simulink model "BLAC_MotorCtrl_Math"  (R2025b)
settings: Solver=FixedStepDiscrete  StartTime=0.0  StopTime=5  FixedStep=MC_Sim_BaseStep  RelTol=1e-3  EnableMultiTasking=on
values from neighbouring files (symbols this model uses):
  MC_Hardware_Chip_ADCResultBit = 0.0    [MotorControlDataDictionary_Math.sldd]
  MC_Hardware_Chip_ADCVoltageMax = 1.0    [MotorControlDataDictionary_Math.sldd]
  MC_Hardware_Chip_ADCVoltageRefence = 0.0    [MotorControlDataDictionary_Math.sldd]
  MC_Hardware_Chip_CSAGain = 1.0    [MotorControlDataDictionary_Math.sldd]
  MC_Sim_BaseStep = 2.5E-8    [MotorControlDataDictionary_Math.sldd]
  MC_Sim_HFTStep = 6.6675E-5    [MotorControlDataDictionary_Math.sldd]
undefined symbols (not defined in the file or in its folder): MC_MOS_DeadTime, MC_Motor_Phi, MC_Motor_Rotor_Pn, MC_Motor_Stator_Ld, MC_Motor_Stator_Lq, MC_Motor_Stator_Rs, MC_Param_CurrentPI_Ki, MC_Param_CurrentPI_Kp, MC_Param_CurrentPI_UdInteMax, MC_Param_CurrentPI_UdInteMin, MC_Param_CurrentPI_UdMax, MC_Param_CurrentPI_UdMin, MC_Param_CurrentPI_UqInteMax, MC_Param_CurrentPI_UqInteMin, MC_Param_CurrentPI_UqMax, MC_Param_CurrentPI_UqMin, MC_Param_Flux_Gamma, MC_Param_Flux_Lalpha, MC_Param_Flux_Lbeta, MC_Param_Flux_Ralpha, MC_Param_Flux_Rbeta, MC_Param_Luen_BEMFalpha, MC_Param_Luen_BEMFbeta, MC_Param_Luen_BEMFErr, MC_Param_Luen_Currentalpha, MC_Param_Luen_Currentbeta, MC_Param_Luen_CurrentErr, MC_Param_Luen_PLL_Ki, MC_Param_Luen_PLL_Kp, MC_Param_Luen_Voltagealpha, MC_Param_Luen_Voltagebeta, MC_Param_PhasetoReal, MC_Param_SMO_CoffA, MC_Param_SMO_CoffB, MC_Param_SpeedtoTheta, MC_Param_SVPWM_DutyMax, MC_Param_SVPWM_DutyMin, MC_Param_SVPWM_SampleOffset1, MC_Param_SVPWM_SampleOffset2, MC_Param_SVPWM_SampleValid
libraries: simulink x31, nesl_utility x22, ee_lib x21, fl_lib x16, spsSeriesRLCBranchLib x2, spsVoltageMeasurementLib x2
(part 3 of 5)

== system BLAC_MotorCtrl_Math/Hardware_Sim/IGBT_Inverter_Sim ==
  DriveA : Inport
  DriveB : Inport  Port=2
  DriveC : Inport  Port=3
  Demux : Demux  Outputs=2
  Demux1 : Demux  Outputs=2
  Demux2 : Demux  Outputs=2
  IGBT_AH : ee_lib/Semiconductors & Converters/IGBT (Ideal, Switching)  port_option=ee.enum.controlport.ps  Vf=0.8 V  Ron=0.001 Ohm  Goff=1e-5 1/Ohm  Vth=6 V  diode_param=ee.enum.semiconductors.protectionDiode.external  diode_Vf=0.8 V  diode_Ron=0.001 Ohm  diode_Goff=1e-5 1/Ohm  diode_C=50e-9 F  diode_iRM=-235 A  diode_iF=300 A  diode_idot=-50 A/us  diode_trr_param=ee.enum.converters.diodeReverseParam.trr_factor  diode_trr_factor=3  diode_trr=15 us  diode_Qrr=1500 s*uA  ice_specify=off  ice_priority=None  ice=0 A  ice_nominal_specify=off  ice_nominal_value=1  ice_nominal_unit=A  vce_specify=off  vce_priority=None  vce=0 V  vce_nominal_specify=off  vce_nominal_value=1  vce_nominal_unit=V  vge_specify=off  vge_priority=None  vge=0 V  vge_nominal_specify=off  vge_nominal_value=1  vge_nominal_unit=V  thermal_loss_option=ee.enum.converters.thermalLossOption.constantvalues  Von_data=[0, .1, .6, .8, 1, 1.3, 1.6, 2, 2.4; 0, .1, .7, 1, 1.2, 1.5, 1.9, 2.4, 2.8] V  Tj=[298.15, 398.15] K  Iout_data=[0, .1, 1, 5, 10, 20, 40, 70, 100] A  Eon_data=[0, .0024, .024, .12, .2, .48, 1.04, 2.16, 3.24; 0, .003, .03, .15, .25, .6, 1.3, 2.7, 4.05] * 1e-3 J  Eoff_data=[0, .0007, .0066, .033, .066, .17, .33, .83, 1.5; 0, .001, .01, .05, .1, .25, .5, 1.2, 2.2] * 1e-3 J  Eon_data_3D=[zeros(2, 9, 3)] J  Eoff_data_3D=[zeros(2, 9, 3)] J  Tj_loss=[298.15, 398.15] K  Iout_data_loss=[0, .1, 1, 5, 10, 20, 40, 70, 100] A  tabulateWithVce=false  Vce_loss=[0, 150, 300] V  Eon_scalar=22.86e-3 J  Eoff_scalar=17.14e-3 J  Voff=300 V  Iout_scalar=600 A  useCurrentFromPreviousCycle=false  useVoltageFromPreviousCycle=false  diodeModelType=ee.enum.converters.diodeModelType.pwl  diodeTableType=ee.enum.diode.tableType.IfMat  diode_ReverseIVType=ee.enum.diode.diodeReverseIV.constant  diode_IfMat=[.07, .12, .19, 1.75, 4.24, 7.32, 11.2; .16, .3, .72, 2.14, 4.02, 6.35, 9.12] A  diode_VfMat=[.9, 1.15, 1.25, 1.5, 1.75, 2.17, 2.6, 2.85; .58, .68, .75, 1.1, 1.38, 1.77, 2.27, 2.7] V  diode_TjVec=[25, 125] degC  diode_VfVec=[.5, .7, .9, 1.3, 1.7, 2.1, 2.5] V  diode_IfVec=[.1, .2, .5, 1, 2, 4, 7, 10] A  diode_IrMat=[1e-06, 2e-06, 5e-06, 1e-05, 2.5e-05, 5e-05, .0001; 2e-06, 5e-06, 1e-05, 4e-05, 8e-05, .0002, .0005] A  diode_VrMat=[10, 100, 200, 250, 300, 325, 350; 10, 70, 160, 220, 270, 300, 320] V  diode_VrVec=[10, 20, 40, 50, 70, 80, 100] V  diode_IrVec=[1e-06, 2e-06, 5e-06, 1e-05, 2e-05, 5e-05, .0001] A  diode_Vr=-600 V  diode_Ls=150 nH  diode_Erec=0.03 J  diode_rec_loss_model=ee.enum.diode.reverseRecoveryModel.fixed  diode_ErecVal=0 J  diode_scaleWithIandV=true  diode_ErecMat=zeros(2, 3) J  diode_TjrecVec=[298.15, 398.15] K  diode_IfrecVec=[.1, 1, 10] A  diode_IrecVal=10 A  diode_VrecVal=10 V  diode_tFilter=1 / 1000 / 100 s  separateThermalPortForDiode=false  thermal_network_parameterization=ee.enum.thermalNetworkTopology.external  Rth=[.08, .5] K/W  Rth_Cauer=[.08, .1, .5] K/W  Rth_Foster=[.08, .14, .22, .16] K/W  thermal_mass_parameterization=ee.enum.thermalNetwork.timeconstant  thermal_mass=[.01, .5] J/K  thermal_mass_Cauer=[.01, .1, .5] J/K  thermal_mass_Foster=[.001, .005, .05, .5] J/K  thermal_time_constant=[.001, .2] s  thermal_time_constant_Cauer=[.001, .1, .2] s  thermal_time_constant_Foster=[7e-05, .0007, .01, .08] s  thermal_mass_initial_temperatures=[25, 25] degC  thermal_mass_initial_temperatures_Cauer=[25, 25, 25] degC  junction_thermal_mass=0.01 J/K  Tvec_initial_Foster=[25, 25, 25, 25] degC  RthDiode=[.03, .2] K/W  RthCauerDiode=[.03, .1, .2] K/W  RthFosterDiode=[.03, .2] K/W  thermalMassDiode=[3, 25] J/K  thermalMassCauerDiode=[3, 10, 25] J/K  thermalMassFosterDiode=[33, 50] J/K  thermalTauDiode=[.1, 5] s  thermalTauCauerDiode=[.1, 1, 5] s  thermalTauFosterDiode=[1, 10] s  thermalMassInitTempDiode=[25, 25] degC  thermalMassInitTempCauerDiode=[25, 25, 25] degC  junctionthermalMassDiode=0.1 J/K  TVecInitialFosterDiode=[25, 25, 25, 25] degC  no_thermal_network=0  IGBT_junction_temperature_specify=off  IGBT_junction_temperature_priority=None  IGBT_junction_temperature=25 degC  IGBT_junction_temperature_nominal_specify=off  IGBT_junction_temperature_nominal_value=1  IGBT_junction_temperature_nominal_unit=degC  diode_junction_temperature_specify=off  diode_junction_temperature_priority=None  diode_junction_temperature=25 degC  diode_junction_temperature_nominal_specify=off  diode_junction_temperature_nominal_value=1  diode_junction_temperature_nominal_unit=degC  Qj_specify=off  Qj_priority=None  Qj=0 W  Qj_nominal_specify=off  Qj_nominal_value=1  Qj_nominal_unit=W  accumulatedSwitchingLosses_specify=off  accumulatedSwitchingLosses_priority=None  accumulatedSwitchingLosses=0 J
  IGBT_AL : ee_lib/Semiconductors & Converters/IGBT (Ideal, Switching)  port_option=ee.enum.controlport.ps  Vf=0.8 V  Ron=0.001 Ohm  Goff=1e-5 1/Ohm  Vth=6 V  diode_param=ee.enum.semiconductors.protectionDiode.external  diode_Vf=0.8 V  diode_Ron=0.001 Ohm  diode_Goff=1e-5 1/Ohm  diode_C=50e-9 F  diode_iRM=-235 A  diode_iF=300 A  diode_idot=-50 A/us  diode_trr_param=ee.enum.converters.diodeReverseParam.trr_factor  diode_trr_factor=3  diode_trr=15 us  diode_Qrr=1500 s*uA  ice_specify=off  ice_priority=None  ice=0 A  ice_nominal_specify=off  ice_nominal_value=1  ice_nominal_unit=A  vce_specify=off  vce_priority=None  vce=0 V  vce_nominal_specify=off  vce_nominal_value=1  vce_nominal_unit=V  vge_specify=off  vge_priority=None  vge=0 V  vge_nominal_specify=off  vge_nominal_value=1  vge_nominal_unit=V  thermal_loss_option=ee.enum.converters.thermalLossOption.constantvalues  Von_data=[0, .1, .6, .8, 1, 1.3, 1.6, 2, 2.4; 0, .1, .7, 1, 1.2, 1.5, 1.9, 2.4, 2.8] V  Tj=[298.15, 398.15] K  Iout_data=[0, .1, 1, 5, 10, 20, 40, 70, 100] A  Eon_data=[0, .0024, .024, .12, .2, .48, 1.04, 2.16, 3.24; 0, .003, .03, .15, .25, .6, 1.3, 2.7, 4.05] * 1e-3 J  Eoff_data=[0, .0007, .0066, .033, .066, .17, .33, .83, 1.5; 0, .001, .01, .05, .1, .25, .5, 1.2, 2.2] * 1e-3 J  Eon_data_3D=[zeros(2, 9, 3)] J  Eoff_data_3D=[zeros(2, 9, 3)] J  Tj_loss=[298.15, 398.15] K  Iout_data_loss=[0, .1, 1, 5, 10, 20, 40, 70, 100] A  tabulateWithVce=false  Vce_loss=[0, 150, 300] V  Eon_scalar=22.86e-3 J  Eoff_scalar=17.14e-3 J  Voff=300 V  Iout_scalar=600 A  useCurrentFromPreviousCycle=false  useVoltageFromPreviousCycle=false  diodeModelType=ee.enum.converters.diodeModelType.pwl  diodeTableType=ee.enum.diode.tableType.IfMat  diode_ReverseIVType=ee.enum.diode.diodeReverseIV.constant  diode_IfMat=[.07, .12, .19, 1.75, 4.24, 7.32, 11.2; .16, .3, .72, 2.14, 4.02, 6.35, 9.12] A  diode_VfMat=[.9, 1.15, 1.25, 1.5, 1.75, 2.17, 2.6, 2.85; .58, .68, .75, 1.1, 1.38, 1.77, 2.27, 2.7] V  diode_TjVec=[25, 125] degC  diode_VfVec=[.5, .7, .9, 1.3, 1.7, 2.1, 2.5] V  diode_IfVec=[.1, .2, .5, 1, 2, 4, 7, 10] A  diode_IrMat=[1e-06, 2e-06, 5e-06, 1e-05, 2.5e-05, 5e-05, .0001; 2e-06, 5e-06, 1e-05, 4e-05, 8e-05, .0002, .0005] A  diode_VrMat=[10, 100, 200, 250, 300, 325, 350; 10, 70, 160, 220, 270, 300, 320] V  diode_VrVec=[10, 20, 40, 50, 70, 80, 100] V  diode_IrVec=[1e-06, 2e-06, 5e-06, 1e-05, 2e-05, 5e-05, .0001] A  diode_Vr=-600 V  diode_Ls=150 nH  diode_Erec=0.03 J  diode_rec_loss_model=ee.enum.diode.reverseRecoveryModel.fixed  diode_ErecVal=0 J  diode_scaleWithIandV=true  diode_ErecMat=zeros(2, 3) J  diode_TjrecVec=[298.15, 398.15] K  diode_IfrecVec=[.1, 1, 10] A  diode_IrecVal=10 A  diode_VrecVal=10 V  diode_tFilter=1 / 1000 / 100 s  separateThermalPortForDiode=false  thermal_network_parameterization=ee.enum.thermalNetworkTopology.external  Rth=[.08, .5] K/W  Rth_Cauer=[.08, .1, .5] K/W  Rth_Foster=[.08, .14, .22, .16] K/W  thermal_mass_parameterization=ee.enum.thermalNetwork.timeconstant  thermal_mass=[.01, .5] J/K  thermal_mass_Cauer=[.01, .1, .5] J/K  thermal_mass_Foster=[.001, .005, .05, .5] J/K  thermal_time_constant=[.001, .2] s  thermal_time_constant_Cauer=[.001, .1, .2] s  thermal_time_constant_Foster=[7e-05, .0007, .01, .08] s  thermal_mass_initial_temperatures=[25, 25] degC  thermal_mass_initial_temperatures_Cauer=[25, 25, 25] degC  junction_thermal_mass=0.01 J/K  Tvec_initial_Foster=[25, 25, 25, 25] degC  RthDiode=[.03, .2] K/W  RthCauerDiode=[.03, .1, .2] K/W  RthFosterDiode=[.03, .2] K/W  thermalMassDiode=[3, 25] J/K  thermalMassCauerDiode=[3, 10, 25] J/K  thermalMassFosterDiode=[33, 50] J/K  thermalTauDiode=[.1, 5] s  thermalTauCauerDiode=[.1, 1, 5] s  thermalTauFosterDiode=[1, 10] s  thermalMassInitTempDiode=[25, 25] degC  thermalMassInitTempCauerDiode=[25, 25, 25] degC  junctionthermalMassDiode=0.1 J/K  TVecInitialFosterDiode=[25, 25, 25, 25] degC  no_thermal_network=0  IGBT_junction_temperature_specify=off  IGBT_junction_temperature_priority=None  IGBT_junction_temperature=25 degC  IGBT_junction_temperature_nominal_specify=off  IGBT_junction_temperature_nominal_value=1  IGBT_junction_temperature_nominal_unit=degC  diode_junction_temperature_specify=off  diode_junction_temperature_priority=None  diode_junction_temperature=25 degC  diode_junction_temperature_nominal_specify=off  diode_junction_temperature_nominal_value=1  diode_junction_temperature_nominal_unit=degC  Qj_specify=off  Qj_priority=None  Qj=0 W  Qj_nominal_specify=off  Qj_nominal_value=1  Qj_nominal_unit=W  accumulatedSwitchingLosses_specify=off  accumulatedSwitchingLosses_priority=None  accumulatedSwitchingLosses=0 J
  IGBT_BH : ee_lib/Semiconductors & Converters/IGBT (Ideal, Switching)  port_option=ee.enum.controlport.ps  Vf=0.8 V  Ron=0.001 Ohm  Goff=1e-5 1/Ohm  Vth=6 V  diode_param=ee.enum.semiconductors.protectionDiode.external  diode_Vf=0.8 V  diode_Ron=0.001 Ohm  diode_Goff=1e-5 1/Ohm  diode_C=50e-9 F  diode_iRM=-235 A  diode_iF=300 A  diode_idot=-50 A/us  diode_trr_param=ee.enum.converters.diodeReverseParam.trr_factor  diode_trr_factor=3  diode_trr=15 us  diode_Qrr=1500 s*uA  ice_specify=off  ice_priority=None  ice=0 A  ice_nominal_specify=off  ice_nominal_value=1  ice_nominal_unit=A  vce_specify=off  vce_priority=None  vce=0 V  vce_nominal_specify=off  vce_nominal_value=1  vce_nominal_unit=V  vge_specify=off  vge_priority=None  vge=0 V  vge_nominal_specify=off  vge_nominal_value=1  vge_nominal_unit=V  thermal_loss_option=ee.enum.converters.thermalLossOption.constantvalues  Von_data=[0, .1, .6, .8, 1, 1.3, 1.6, 2, 2.4; 0, .1, .7, 1, 1.2, 1.5, 1.9, 2.4, 2.8] V  Tj=[298.15, 398.15] K  Iout_data=[0, .1, 1, 5, 10, 20, 40, 70, 100] A  Eon_data=[0, .0024, .024, .12, .2, .48, 1.04, 2.16, 3.24; 0, .003, .03, .15, .25, .6, 1.3, 2.7, 4.05] * 1e-3 J  Eoff_data=[0, .0007, .0066, .033, .066, .17, .33, .83, 1.5; 0, .001, .01, .05, .1, .25, .5, 1.2, 2.2] * 1e-3 J  Eon_data_3D=[zeros(2, 9, 3)] J  Eoff_data_3D=[zeros(2, 9, 3)] J  Tj_loss=[298.15, 398.15] K  Iout_data_loss=[0, .1, 1, 5, 10, 20, 40, 70, 100] A  tabulateWithVce=false  Vce_loss=[0, 150, 300] V  Eon_scalar=22.86e-3 J  Eoff_scalar=17.14e-3 J  Voff=300 V  Iout_scalar=600 A  useCurrentFromPreviousCycle=false  useVoltageFromPreviousCycle=false  diodeModelType=ee.enum.converters.diodeModelType.pwl  diodeTableType=ee.enum.diode.tableType.IfMat  diode_ReverseIVType=ee.enum.diode.diodeReverseIV.constant  diode_IfMat=[.07, .12, .19, 1.75, 4.24, 7.32, 11.2; .16, .3, .72, 2.14, 4.02, 6.35, 9.12] A  diode_VfMat=[.9, 1.15, 1.25, 1.5, 1.75, 2.17, 2.6, 2.85; .58, .68, .75, 1.1, 1.38, 1.77, 2.27, 2.7] V  diode_TjVec=[25, 125] degC  diode_VfVec=[.5, .7, .9, 1.3, 1.7, 2.1, 2.5] V  diode_IfVec=[.1, .2, .5, 1, 2, 4, 7, 10] A  diode_IrMat=[1e-06, 2e-06, 5e-06, 1e-05, 2.5e-05, 5e-05, .0001; 2e-06, 5e-06, 1e-05, 4e-05, 8e-05, .0002, .0005] A  diode_VrMat=[10, 100, 200, 250, 300, 325, 350; 10, 70, 160, 220, 270, 300, 320] V  diode_VrVec=[10, 20, 40, 50, 70, 80, 100] V  diode_IrVec=[1e-06, 2e-06, 5e-06, 1e-05, 2e-05, 5e-05, .0001] A  diode_Vr=-600 V  diode_Ls=150 nH  diode_Erec=0.03 J  diode_rec_loss_model=ee.enum.diode.reverseRecoveryModel.fixed  diode_ErecVal=0 J  diode_scaleWithIandV=true  diode_ErecMat=zeros(2, 3) J  diode_TjrecVec=[298.15, 398.15] K  diode_IfrecVec=[.1, 1, 10] A  diode_IrecVal=10 A  diode_VrecVal=10 V  diode_tFilter=1 / 1000 / 100 s  separateThermalPortForDiode=false  thermal_network_parameterization=ee.enum.thermalNetworkTopology.external  Rth=[.08, .5] K/W  Rth_Cauer=[.08, .1, .5] K/W  Rth_Foster=[.08, .14, .22, .16] K/W  thermal_mass_parameterization=ee.enum.thermalNetwork.timeconstant  thermal_mass=[.01, .5] J/K  thermal_mass_Cauer=[.01, .1, .5] J/K  thermal_mass_Foster=[.001, .005, .05, .5] J/K  thermal_time_constant=[.001, .2] s  thermal_time_constant_Cauer=[.001, .1, .2] s  thermal_time_constant_Foster=[7e-05, .0007, .01, .08] s  thermal_mass_initial_temperatures=[25, 25] degC  thermal_mass_initial_temperatures_Cauer=[25, 25, 25] degC  junction_thermal_mass=0.01 J/K  Tvec_initial_Foster=[25, 25, 25, 25] degC  RthDiode=[.03, .2] K/W  RthCauerDiode=[.03, .1, .2] K/W  RthFosterDiode=[.03, .2] K/W  thermalMassDiode=[3, 25] J/K  thermalMassCauerDiode=[3, 10, 25] J/K  thermalMassFosterDiode=[33, 50] J/K  thermalTauDiode=[.1, 5] s  thermalTauCauerDiode=[.1, 1, 5] s  thermalTauFosterDiode=[1, 10] s  thermalMassInitTempDiode=[25, 25] degC  thermalMassInitTempCauerDiode=[25, 25, 25] degC  junctionthermalMassDiode=0.1 J/K  TVecInitialFosterDiode=[25, 25, 25, 25] degC  no_thermal_network=0  IGBT_junction_temperature_specify=off  IGBT_junction_temperature_priority=None  IGBT_junction_temperature=25 degC  IGBT_junction_temperature_nominal_specify=off  IGBT_junction_temperature_nominal_value=1  IGBT_junction_temperature_nominal_unit=degC  diode_junction_temperature_specify=off  diode_junction_temperature_priority=None  diode_junction_temperature=25 degC  diode_junction_temperature_nominal_specify=off  diode_junction_temperature_nominal_value=1  diode_junction_temperature_nominal_unit=degC  Qj_specify=off  Qj_priority=None  Qj=0 W  Qj_nominal_specify=off  Qj_nominal_value=1  Qj_nominal_unit=W  accumulatedSwitchingLosses_specify=off  accumulatedSwitchingLosses_priority=None  accumulatedSwitchingLosses=0 J
  IGBT_BL : ee_lib/Semiconductors & Converters/IGBT (Ideal, Switching)  port_option=ee.enum.controlport.ps  Vf=0.8 V  Ron=0.001 Ohm  Goff=1e-5 1/Ohm  Vth=6 V  diode_param=ee.enum.semiconductors.protectionDiode.external  diode_Vf=0.8 V  diode_Ron=0.001 Ohm  diode_Goff=1e-5 1/Ohm  diode_C=50e-9 F  diode_iRM=-235 A  diode_iF=300 A  diode_idot=-50 A/us  diode_trr_param=ee.enum.converters.diodeReverseParam.trr_factor  diode_trr_factor=3  diode_trr=15 us  diode_Qrr=1500 s*uA  ice_specify=off  ice_priority=None  ice=0 A  ice_nominal_specify=off  ice_nominal_value=1  ice_nominal_unit=A  vce_specify=off  vce_priority=None  vce=0 V  vce_nominal_specify=off  vce_nominal_value=1  vce_nominal_unit=V  vge_specify=off  vge_priority=None  vge=0 V  vge_nominal_specify=off  vge_nominal_value=1  vge_nominal_unit=V  thermal_loss_option=ee.enum.converters.thermalLossOption.constantvalues  Von_data=[0, .1, .6, .8, 1, 1.3, 1.6, 2, 2.4; 0, .1, .7, 1, 1.2, 1.5, 1.9, 2.4, 2.8] V  Tj=[298.15, 398.15] K  Iout_data=[0, .1, 1, 5, 10, 20, 40, 70, 100] A  Eon_data=[0, .0024, .024, .12, .2, .48, 1.04, 2.16, 3.24; 0, .003, .03, .15, .25, .6, 1.3, 2.7, 4.05] * 1e-3 J  Eoff_data=[0, .0007, .0066, .033, .066, .17, .33, .83, 1.5; 0, .001, .01, .05, .1, .25, .5, 1.2, 2.2] * 1e-3 J  Eon_data_3D=[zeros(2, 9, 3)] J  Eoff_data_3D=[zeros(2, 9, 3)] J  Tj_loss=[298.15, 398.15] K  Iout_data_loss=[0, .1, 1, 5, 10, 20, 40, 70, 100] A  tabulateWithVce=false  Vce_loss=[0, 150, 300] V  Eon_scalar=22.86e-3 J  Eoff_scalar=17.14e-3 J  Voff=300 V  Iout_scalar=600 A  useCurrentFromPreviousCycle=false  useVoltageFromPreviousCycle=false  diodeModelType=ee.enum.converters.diodeModelType.pwl  diodeTableType=ee.enum.diode.tableType.IfMat  diode_ReverseIVType=ee.enum.diode.diodeReverseIV.constant  diode_IfMat=[.07, .12, .19, 1.75, 4.24, 7.32, 11.2; .16, .3, .72, 2.14, 4.02, 6.35, 9.12] A  diode_VfMat=[.9, 1.15, 1.25, 1.5, 1.75, 2.17, 2.6, 2.85; .58, .68, .75, 1.1, 1.38, 1.77, 2.27, 2.7] V  diode_TjVec=[25, 125] degC  diode_VfVec=[.5, .7, .9, 1.3, 1.7, 2.1, 2.5] V  diode_IfVec=[.1, .2, .5, 1, 2, 4, 7, 10] A  diode_IrMat=[1e-06, 2e-06, 5e-06, 1e-05, 2.5e-05, 5e-05, .0001; 2e-06, 5e-06, 1e-05, 4e-05, 8e-05, .0002, .0005] A  diode_VrMat=[10, 100, 200, 250, 300, 325, 350; 10, 70, 160, 220, 270, 300, 320] V  diode_VrVec=[10, 20, 40, 50, 70, 80, 100] V  diode_IrVec=[1e-06, 2e-06, 5e-06, 1e-05, 2e-05, 5e-05, .0001] A  diode_Vr=-600 V  diode_Ls=150 nH  diode_Erec=0.03 J  diode_rec_loss_model=ee.enum.diode.reverseRecoveryModel.fixed  diode_ErecVal=0 J  diode_scaleWithIandV=true  diode_ErecMat=zeros(2, 3) J  diode_TjrecVec=[298.15, 398.15] K  diode_IfrecVec=[.1, 1, 10] A  diode_IrecVal=10 A  diode_VrecVal=10 V  diode_tFilter=1 / 1000 / 100 s  separateThermalPortForDiode=false  thermal_network_parameterization=ee.enum.thermalNetworkTopology.external  Rth=[.08, .5] K/W  Rth_Cauer=[.08, .1, .5] K/W  Rth_Foster=[.08, .14, .22, .16] K/W  thermal_mass_parameterization=ee.enum.thermalNetwork.timeconstant  thermal_mass=[.01, .5] J/K  thermal_mass_Cauer=[.01, .1, .5] J/K  thermal_mass_Foster=[.001, .005, .05, .5] J/K  thermal_time_constant=[.001, .2] s  thermal_time_constant_Cauer=[.001, .1, .2] s  thermal_time_constant_Foster=[7e-05, .0007, .01, .08] s  thermal_mass_initial_temperatures=[25, 25] degC  thermal_mass_initial_temperatures_Cauer=[25, 25, 25] degC  junction_thermal_mass=0.01 J/K  Tvec_initial_Foster=[25, 25, 25, 25] degC  RthDiode=[.03, .2] K/W  RthCauerDiode=[.03, .1, .2] K/W  RthFosterDiode=[.03, .2] K/W  thermalMassDiode=[3, 25] J/K  thermalMassCauerDiode=[3, 10, 25] J/K  thermalMassFosterDiode=[33, 50] J/K  thermalTauDiode=[.1, 5] s  thermalTauCauerDiode=[.1, 1, 5] s  thermalTauFosterDiode=[1, 10] s  thermalMassInitTempDiode=[25, 25] degC  thermalMassInitTempCauerDiode=[25, 25, 25] degC  junctionthermalMassDiode=0.1 J/K  TVecInitialFosterDiode=[25, 25, 25, 25] degC  no_thermal_network=0  IGBT_junction_temperature_specify=off  IGBT_junction_temperature_priority=None  IGBT_junction_temperature=25 degC  IGBT_junction_temperature_nominal_specify=off  IGBT_junction_temperature_nominal_value=1  IGBT_junction_temperature_nominal_unit=degC  diode_junction_temperature_specify=off  diode_junction_temperature_priority=None  diode_junction_temperature=25 degC  diode_junction_temperature_nominal_specify=off  diode_junction_temperature_nominal_value=1  diode_junction_temperature_nominal_unit=degC  Qj_specify=off  Qj_priority=None  Qj=0 W  Qj_nominal_specify=off  Qj_nominal_value=1  Qj_nominal_unit=W  accumulatedSwitchingLosses_specify=off  accumulatedSwitchingLosses_priority=None  accumulatedSwitchingLosses=0 J
  IGBT_CH : ee_lib/Semiconductors & Converters/IGBT (Ideal, Switching)  port_option=ee.enum.controlport.ps  Vf=0.8 V  Ron=0.001 Ohm  Goff=1e-5 1/Ohm  Vth=6 V  diode_param=ee.enum.semiconductors.protectionDiode.external  diode_Vf=0.8 V  diode_Ron=0.001 Ohm  diode_Goff=1e-5 1/Ohm  diode_C=50e-9 F  diode_iRM=-235 A  diode_iF=300 A  diode_idot=-50 A/us  diode_trr_param=ee.enum.converters.diodeReverseParam.trr_factor  diode_trr_factor=3  diode_trr=15 us  diode_Qrr=1500 s*uA  ice_specify=off  ice_priority=None  ice=0 A  ice_nominal_specify=off  ice_nominal_value=1  ice_nominal_unit=A  vce_specify=off  vce_priority=None  vce=0 V  vce_nominal_specify=off  vce_nominal_value=1  vce_nominal_unit=V  vge_specify=off  vge_priority=None  vge=0 V  vge_nominal_specify=off  vge_nominal_value=1  vge_nominal_unit=V  thermal_loss_option=ee.enum.converters.thermalLossOption.constantvalues  Von_data=[0, .1, .6, .8, 1, 1.3, 1.6, 2, 2.4; 0, .1, .7, 1, 1.2, 1.5, 1.9, 2.4, 2.8] V  Tj=[298.15, 398.15] K  Iout_data=[0, .1, 1, 5, 10, 20, 40, 70, 100] A  Eon_data=[0, .0024, .024, .12, .2, .48, 1.04, 2.16, 3.24; 0, .003, .03, .15, .25, .6, 1.3, 2.7, 4.05] * 1e-3 J  Eoff_data=[0, .0007, .0066, .033, .066, .17, .33, .83, 1.5; 0, .001, .01, .05, .1, .25, .5, 1.2, 2.2] * 1e-3 J  Eon_data_3D=[zeros(2, 9, 3)] J  Eoff_data_3D=[zeros(2, 9, 3)] J  Tj_loss=[298.15, 398.15] K  Iout_data_loss=[0, .1, 1, 5, 10, 20, 40, 70, 100] A  tabulateWithVce=false  Vce_loss=[0, 150, 300] V  Eon_scalar=22.86e-3 J  Eoff_scalar=17.14e-3 J  Voff=300 V  Iout_scalar=600 A  useCurrentFromPreviousCycle=false  useVoltageFromPreviousCycle=false  diodeModelType=ee.enum.converters.diodeModelType.pwl  diodeTableType=ee.enum.diode.tableType.IfMat  diode_ReverseIVType=ee.enum.diode.diodeReverseIV.constant  diode_IfMat=[.07, .12, .19, 1.75, 4.24, 7.32, 11.2; .16, .3, .72, 2.14, 4.02, 6.35, 9.12] A  diode_VfMat=[.9, 1.15, 1.25, 1.5, 1.75, 2.17, 2.6, 2.85; .58, .68, .75, 1.1, 1.38, 1.77, 2.27, 2.7] V  diode_TjVec=[25, 125] degC  diode_VfVec=[.5, .7, .9, 1.3, 1.7, 2.1, 2.5] V  diode_IfVec=[.1, .2, .5, 1, 2, 4, 7, 10] A  diode_IrMat=[1e-06, 2e-06, 5e-06, 1e-05, 2.5e-05, 5e-05, .0001; 2e-06, 5e-06, 1e-05, 4e-05, 8e-05, .0002, .0005] A  diode_VrMat=[10, 100, 200, 250, 300, 325, 350; 10, 70, 160, 220, 270, 300, 320] V  diode_VrVec=[10, 20, 40, 50, 70, 80, 100] V  diode_IrVec=[1e-06, 2e-06, 5e-06, 1e-05, 2e-05, 5e-05, .0001] A  diode_Vr=-600 V  diode_Ls=150 nH  diode_Erec=0.03 J  diode_rec_loss_model=ee.enum.diode.reverseRecoveryModel.fixed  diode_ErecVal=0 J  diode_scaleWithIandV=true  diode_ErecMat=zeros(2, 3) J  diode_TjrecVec=[298.15, 398.15] K  diode_IfrecVec=[.1, 1, 10] A  diode_IrecVal=10 A  diode_VrecVal=10 V  diode_tFilter=1 / 1000 / 100 s  separateThermalPortForDiode=false  thermal_network_parameterization=ee.enum.thermalNetworkTopology.external  Rth=[.08, .5] K/W  Rth_Cauer=[.08, .1, .5] K/W  Rth_Foster=[.08, .14, .22, .16] K/W  thermal_mass_parameterization=ee.enum.thermalNetwork.timeconstant  thermal_mass=[.01, .5] J/K  thermal_mass_Cauer=[.01, .1, .5] J/K  thermal_mass_Foster=[.001, .005, .05, .5] J/K  thermal_time_constant=[.001, .2] s  thermal_time_constant_Cauer=[.001, .1, .2] s  thermal_time_constant_Foster=[7e-05, .0007, .01, .08] s  thermal_mass_initial_temperatures=[25, 25] degC  thermal_mass_initial_temperatures_Cauer=[25, 25, 25] degC  junction_thermal_mass=0.01 J/K  Tvec_initial_Foster=[25, 25, 25, 25] degC  RthDiode=[.03, .2] K/W  RthCauerDiode=[.03, .1, .2] K/W  RthFosterDiode=[.03, .2] K/W  thermalMassDiode=[3, 25] J/K  thermalMassCauerDiode=[3, 10, 25] J/K  thermalMassFosterDiode=[33, 50] J/K  thermalTauDiode=[.1, 5] s  thermalTauCauerDiode=[.1, 1, 5] s  thermalTauFosterDiode=[1, 10] s  thermalMassInitTempDiode=[25, 25] degC  thermalMassInitTempCauerDiode=[25, 25, 25] degC  junctionthermalMassDiode=0.1 J/K  TVecInitialFosterDiode=[25, 25, 25, 25] degC  no_thermal_network=0  IGBT_junction_temperature_specify=off  IGBT_junction_temperature_priority=None  IGBT_junction_temperature=25 degC  IGBT_junction_temperature_nominal_specify=off  IGBT_junction_temperature_nominal_value=1  IGBT_junction_temperature_nominal_unit=degC  diode_junction_temperature_specify=off  diode_junction_temperature_priority=None  diode_junction_temperature=25 degC  diode_junction_temperature_nominal_specify=off  diode_junction_temperature_nominal_value=1  diode_junction_temperature_nominal_unit=degC  Qj_specify=off  Qj_priority=None  Qj=0 W  Qj_nominal_specify=off  Qj_nominal_value=1  Qj_nominal_unit=W  accumulatedSwitchingLosses_specify=off  accumulatedSwitchingLosses_priority=None  accumulatedSwitchingLosses=0 J
  IGBT_CL : ee_lib/Semiconductors & Converters/IGBT (Ideal, Switching)  port_option=ee.enum.controlport.ps  Vf=0.8 V  Ron=0.001 Ohm  Goff=1e-5 1/Ohm  Vth=6 V  diode_param=ee.enum.semiconductors.protectionDiode.external  diode_Vf=0.8 V  diode_Ron=0.001 Ohm  diode_Goff=1e-5 1/Ohm  diode_C=50e-9 F  diode_iRM=-235 A  diode_iF=300 A  diode_idot=-50 A/us  diode_trr_param=ee.enum.converters.diodeReverseParam.trr_factor  diode_trr_factor=3  diode_trr=15 us  diode_Qrr=1500 s*uA  ice_specify=off  ice_priority=None  ice=0 A  ice_nominal_specify=off  ice_nominal_value=1  ice_nominal_unit=A  vce_specify=off  vce_priority=None  vce=0 V  vce_nominal_specify=off  vce_nominal_value=1  vce_nominal_unit=V  vge_specify=off  vge_priority=None  vge=0 V  vge_nominal_specify=off  vge_nominal_value=1  vge_nominal_unit=V  thermal_loss_option=ee.enum.converters.thermalLossOption.constantvalues  Von_data=[0, .1, .6, .8, 1, 1.3, 1.6, 2, 2.4; 0, .1, .7, 1, 1.2, 1.5, 1.9, 2.4, 2.8] V  Tj=[298.15, 398.15] K  Iout_data=[0, .1, 1, 5, 10, 20, 40, 70, 100] A  Eon_data=[0, .0024, .024, .12, .2, .48, 1.04, 2.16, 3.24; 0, .003, .03, .15, .25, .6, 1.3, 2.7, 4.05] * 1e-3 J  Eoff_data=[0, .0007, .0066, .033, .066, .17, .33, .83, 1.5; 0, .001, .01, .05, .1, .25, .5, 1.2, 2.2] * 1e-3 J  Eon_data_3D=[zeros(2, 9, 3)] J  Eoff_data_3D=[zeros(2, 9, 3)] J  Tj_loss=[298.15, 398.15] K  Iout_data_loss=[0, .1, 1, 5, 10, 20, 40, 70, 100] A  tabulateWithVce=false  Vce_loss=[0, 150, 300] V  Eon_scalar=22.86e-3 J  Eoff_scalar=17.14e-3 J  Voff=300 V  Iout_scalar=600 A  useCurrentFromPreviousCycle=false  useVoltageFromPreviousCycle=false  diodeModelType=ee.enum.converters.diodeModelType.pwl  diodeTableType=ee.enum.diode.tableType.IfMat  diode_ReverseIVType=ee.enum.diode.diodeReverseIV.constant  diode_IfMat=[.07, .12, .19, 1.75, 4.24, 7.32, 11.2; .16, .3, .72, 2.14, 4.02, 6.35, 9.12] A  diode_VfMat=[.9, 1.15, 1.25, 1.5, 1.75, 2.17, 2.6, 2.85; .58, .68, .75, 1.1, 1.38, 1.77, 2.27, 2.7] V  diode_TjVec=[25, 125] degC  diode_VfVec=[.5, .7, .9, 1.3, 1.7, 2.1, 2.5] V  diode_IfVec=[.1, .2, .5, 1, 2, 4, 7, 10] A  diode_IrMat=[1e-06, 2e-06, 5e-06, 1e-05, 2.5e-05, 5e-05, .0001; 2e-06, 5e-06, 1e-05, 4e-05, 8e-05, .0002, .0005] A  diode_VrMat=[10, 100, 200, 250, 300, 325, 350; 10, 70, 160, 220, 270, 300, 320] V  diode_VrVec=[10, 20, 40, 50, 70, 80, 100] V  diode_IrVec=[1e-06, 2e-06, 5e-06, 1e-05, 2e-05, 5e-05, .0001] A  diode_Vr=-600 V  diode_Ls=150 nH  diode_Erec=0.03 J  diode_rec_loss_model=ee.enum.diode.reverseRecoveryModel.fixed  diode_ErecVal=0 J  diode_scaleWithIandV=true  diode_ErecMat=zeros(2, 3) J  diode_TjrecVec=[298.15, 398.15] K  diode_IfrecVec=[.1, 1, 10] A  diode_IrecVal=10 A  diode_VrecVal=10 V  diode_tFilter=1 / 1000 / 100 s  separateThermalPortForDiode=false  thermal_network_parameterization=ee.enum.thermalNetworkTopology.external  Rth=[.08, .5] K/W  Rth_Cauer=[.08, .1, .5] K/W  Rth_Foster=[.08, .14, .22, .16] K/W  thermal_mass_parameterization=ee.enum.thermalNetwork.timeconstant  thermal_mass=[.01, .5] J/K  thermal_mass_Cauer=[.01, .1, .5] J/K  thermal_mass_Foster=[.001, .005, .05, .5] J/K  thermal_time_constant=[.001, .2] s  thermal_time_constant_Cauer=[.001, .1, .2] s  thermal_time_constant_Foster=[7e-05, .0007, .01, .08] s  thermal_mass_initial_temperatures=[25, 25] degC  thermal_mass_initial_temperatures_Cauer=[25, 25, 25] degC  junction_thermal_mass=0.01 J/K  Tvec_initial_Foster=[25, 25, 25, 25] degC  RthDiode=[.03, .2] K/W  RthCauerDiode=[.03, .1, .2] K/W  RthFosterDiode=[.03, .2] K/W  thermalMassDiode=[3, 25] J/K  thermalMassCauerDiode=[3, 10, 25] J/K  thermalMassFosterDiode=[33, 50] J/K  thermalTauDiode=[.1, 5] s  thermalTauCauerDiode=[.1, 1, 5] s  thermalTauFosterDiode=[1, 10] s  thermalMassInitTempDiode=[25, 25] degC  thermalMassInitTempCauerDiode=[25, 25, 25] degC  junctionthermalMassDiode=0.1 J/K  TVecInitialFosterDiode=[25, 25, 25, 25] degC  no_thermal_network=0  IGBT_junction_temperature_specify=off  IGBT_junction_temperature_priority=None  IGBT_junction_temperature=25 degC  IGBT_junction_temperature_nominal_specify=off  IGBT_junction_temperature_nominal_value=1  IGBT_junction_temperature_nominal_unit=degC  diode_junction_temperature_specify=off  diode_junction_temperature_priority=None  diode_junction_temperature=25 degC  diode_junction_temperature_nominal_specify=off  diode_junction_temperature_nominal_value=1  diode_junction_temperature_nominal_unit=degC  Qj_specify=off  Qj_priority=None  Qj=0 W  Qj_nominal_specify=off  Qj_nominal_value=1  Qj_nominal_unit=W  accumulatedSwitchingLosses_specify=off  accumulatedSwitchingLosses_priority=None  accumulatedSwitchingLosses=0 J
  Simulink-PS Converter{,1..5} (6 alike) : nesl_utility/Simulink-PS Converter  PhysicalDomain=network_engine_domain  SubClassName=ps_input  LeftPortType=input  RightPortType=output  PseudoPeriodic=off  Frequencies=[]  NoiseDistribution=none  NoiseParameters=[]  Unit=1  AffineConversion=off  FilteringAndDerivatives=provide  SimscapeFilterOrder=1  InputFilterTimeConstant=0.001  UdotUserProvided=0
  Vdc : PMIOPort  Side=Left
  A : PMIOPort  Port=2  Side=Right
  B : PMIOPort  Port=3  Side=Right
  C : PMIOPort  Port=4  Side=Right
  AL : PMIOPort  Port=5  Side=Right
  BL : PMIOPort  Port=6  Side=Right
  CL : PMIOPort  Port=7  Side=Right
  wires:
  [Drive_BL] -> Simulink-PS Converter3/1
  DriveC/1 -> Demux2/1
  Demux/2 -> [Drive_AL]
  DriveA/1 -> Demux/1
  Demux1/1 -> [Drive_BH]
  [Drive_BH] -> Simulink-PS Converter2/1
  Demux2/1 -> [Drive_CH]
  DriveB/1 -> Demux1/1
  Demux/1 -> [Drive_AH]
  [Drive_AL] -> Simulink-PS Converter1/1
  [Drive_CL] -> Simulink-PS Converter4/1
  [Drive_CH] -> Simulink-PS Converter5/1
  Demux2/2 -> [Drive_CL]
  Demux1/2 -> [Drive_BL]
  [Drive_AH] -> Simulink-PS Converter/1
  connections:
  IGBT_AH/RConn1 -- IGBT_CH/RConn1 -- IGBT_BH/RConn1 -- Vdc/RConn1
  Simulink-PS Converter3/RConn1 -- IGBT_BL/LConn1
  Simulink-PS Converter1/RConn1 -- IGBT_AL/LConn1
  IGBT_CL/RConn2 -- CL/RConn1
  Simulink-PS Converter/RConn1 -- IGBT_AH/LConn1
  IGBT_BL/RConn2 -- BL/RConn1
  IGBT_BH/RConn2 -- B/RConn1 -- IGBT_BL/RConn1
  Simulink-PS Converter5/RConn1 -- IGBT_CH/LConn1
  IGBT_CH/RConn2 -- C/RConn1 -- IGBT_CL/RConn1
  IGBT_AH/RConn2 -- A/RConn1 -- IGBT_AL/RConn1
  Simulink-PS Converter2/RConn1 -- IGBT_BH/LConn1
  IGBT_AL/RConn2 -- AL/RConn1
  Simulink-PS Converter4/RConn1 -- IGBT_CL/LConn1

== system BLAC_MotorCtrl_Math/Hardware_Sim/Motor_Machine_Sim ==
  LoadTorque : Inport
  Bus Creator : BusCreator  Inputs=4
  Ideal Rotational Motion Sensor : fl_lib/Mechanical/Mechanical Sensors/Ideal Rotational Motion Sensor  reference=foundation.enum.MeasurementReference.difference  acceleration_port=true  velocity_port=true  position_port=true  wrap_angle=true  offset=0 rad
      settings: InternalSimscapePortConfiguration="{\"Bottom\":[],\"Left\":[{\"id\":\"R\",\"label\":\"R\",\"type\":\"foundation.mechanical.rotational.rotational\"}],\"Right\":[{\"id\":\"C\",\"label\":\"C\",\"type\":\"foundation.mechanical.rotational.rotational\"},{\"id\":\"alpha\",\"label\":\"α\",\"type\":\"output\"},{\"id\":\"W\",\"label\":\"W\",\"type\":\"output\"},{\"id\":\"A\",\"label\":\"A\",\"type\":\"output\"}],\"Top\":[]}"
  Ideal Torque Sensor : fl_lib/Mechanical/Mechanical Sensors/Ideal Torque Sensor
  Ideal Torque Source : fl_lib/Mechanical/Mechanical Sources/Ideal Torque Source
  Inertia : fl_lib/Mechanical/Rotational Elements/Inertia  inertia=0.01 kg*m^2  num_ports=foundation.enum.numPorts2.one  w_specify=off  w_priority=High  w=0 rad/s  w_nominal_specify=off  w_nominal_value=1  w_nominal_unit=rad/s  t_specify=off  t_priority=None  t=0 N*m  t_nominal_specify=off  t_nominal_value=1  t_nominal_unit=N*m
  Mechanical Rotational Reference : fl_lib/Mechanical/Rotational Elements/Mechanical Rotational Reference
  PS-Simulink Converter{,1..3} (4 alike) : nesl_utility/PS-Simulink Converter  PhysicalDomain=network_engine_domain  SubClassName=ps_output  LeftPortType=input  RightPortType=output  PseudoPeriodic=off  Frequencies=[]  VectorFormat=inherit  Unit=inherit  AffineConversion=off
  Simulink-PS Converter : nesl_utility/Simulink-PS Converter  PhysicalDomain=network_engine_domain  SubClassName=ps_input  LeftPortType=input  RightPortType=output  PseudoPeriodic=off  Frequencies=[]  NoiseDistribution=none  NoiseParameters=[]  Unit=1  AffineConversion=off  FilteringAndDerivatives=provide  SimscapeFilterOrder=1  InputFilterTimeConstant=0.001  UdotUserProvided=0
  R : PMIOPort  Side=Left
  C : PMIOPort  Port=2  Side=Left
  MachineM : Outport
  wires:
  LoadTorque/1 -> Simulink-PS Converter/1
  PS-Simulink Converter2/1 -> Bus Creator/4  "Tm"
  PS-Simulink Converter1/1 -> Bus Creator/3  "ThetaM"
  PS-Simulink Converter/1 -> Bus Creator/2  "Wm"
  PS-Simulink Converter3/1 -> Bus Creator/1  "Acceleration"
  Bus Creator/1 -> MachineM/1  "MachineM"
  connections:
  R/RConn1 -- Ideal Torque Source/LConn1 -- Ideal Rotational Motion Sensor/LConn1 -- Inertia/LConn1 -- Ideal Torque Sensor/LConn1
  C/RConn1 -- Ideal Rotational Motion Sensor/RConn1 -- Ideal Torque Sensor/RConn1 -- Ideal Torque Source/RConn2 -- Mechanical Rotational Reference/LConn1
  PS-Simulink Converter2/LConn1 -- Ideal Torque Sensor/RConn2
  PS-Simulink Converter1/LConn1 -- Ideal Rotational Motion Sensor/RConn4
  PS-Simulink Converter/LConn1 -- Ideal Rotational Motion Sensor/RConn3
  PS-Simulink Converter3/LConn1 -- Ideal Rotational Motion Sensor/RConn2
  Ideal Torque Source/RConn1 -- Simulink-PS Converter/RConn1

== system BLAC_MotorCtrl_Math/Hardware_Sim/SampleTrigger_Sim ==
  ClockCounter : Inport
  SamplePoint : Inport  Port=2
  Data Type Conversion{,1..4} (5 alike) : DataTypeConversion  OutDataTypeStr=double  RndMeth=Simplest  SaturateOnIntegerOverflow=off
  Demux : Demux  Outputs=5
  Mux : Mux  Inputs=3
  Relational Operator{,1..4} (5 alike) : RelationalOperator  Operator=>  OutDataTypeStr=boolean  RndMeth=Simplest  InputSameDT=off
  Current_Sample_Trigger : Outport
  Vbus_Sample_Trigger : Outport  Port=2
  Temp_Sample_Trigger : Outport  Port=3
  wires:
  SamplePoint/1 -> Demux/1
  Relational Operator/1 -> Data Type Conversion/1
  Demux/1 -> Relational Operator/2
  Demux/2 -> Relational Operator1/2
  Relational Operator1/1 -> Data Type Conversion1/1
  Relational Operator2/1 -> Data Type Conversion2/1
  Demux/4 -> Relational Operator2/2
  Demux/5 -> Relational Operator3/2
  Relational Operator3/1 -> Data Type Conversion3/1
  ClockCounter/1 -> Relational Operator4/1, Relational Operator3/1, Relational Operator2/1, Relational Operator1/1, Relational Operator/1
  Data Type Conversion/1 -> Mux/1
  Data Type Conversion1/1 -> Mux/2
  Mux/1 -> Current_Sample_Trigger/1
  Data Type Conversion2/1 -> Vbus_Sample_Trigger/1
  Data Type Conversion3/1 -> Temp_Sample_Trigger/1
  Demux/3 -> Relational Operator4/2
  Relational Operator4/1 -> Data Type Conversion4/1
  Data Type Conversion4/1 -> Mux/3

== system BLAC_MotorCtrl_Math/Hardware_Sim/Subsystem ==
  Mux : Mux  Inputs=2
  Mux1 : Mux  Inputs=2
  Mux2 : Mux  Inputs=2
  PhaseM : Subsystem
  PhaseM1 : Subsystem
  PhaseM2 : Subsystem
  Resistor : ee_lib/Passive/Resistor  R=1 Ohm  enable_R_tol=ee.enum.toleranceApplication.none  R_tol=5  tol_distribution=ee.enum.toleranceDistribution.uniform  nSigma=4  enable_operating_limits=ee.enum.enable.no  operating_limit_action=ee.enum.passive.reportOpLim.warn  power_rating=1 W  max_working_voltage=100 V  noise_mode=ee.enum.sources.noise.Disabled  Tdevice=25 degC  sample_time=1e-3 s  repeatability=ee.enum.ic.repeatability.notRepeatable  user_seed=0  auto_seed=2084672538  power_derating_T1=70 degC  power_derating_T2=155 degC  operating_temperature_range_vec=[-50, 150] degC  alpha=3.93e-3 1/K  Tmeas=25 degC  thermal_mass=100 J/K  temperature_specify=off  temperature_priority=High  temperature=298.15 K  temperature_nominal_specify=off  temperature_nominal_value=1  temperature_nominal_unit=K
  PhaseInputA : PMIOPort  Side=Left
  PhaseInputB : PMIOPort  Port=2  Side=Left
  PhaseInputC : PMIOPort  Port=3  Side=Left
  PhaseOutA : PMIOPort  Port=4  Side=Right
  PhaseOutB : PMIOPort  Port=5  Side=Right
  PhaseOutC : PMIOPort  Port=6  Side=Right
  N : PMIOPort  Port=7  Side=Right
  GND : PMIOPort  Port=8  Side=Right
  PhaseAM : Outport
  PhaseBM : Outport  Port=2
  PhaseCM : Outport  Port=3
  wires:
  Mux1/1 -> [PhaseBM]
  PhaseM/1(PhaseCurrent) -> Mux/1
  PhaseM2/2(PhaseVoltage) -> Mux2/2
  PhaseM/2(PhaseVoltage) -> Mux/2
  PhaseM2/1(PhaseCurrent) -> Mux2/1
  PhaseM1/2(PhaseVoltage) -> Mux1/2
  PhaseM1/1(PhaseCurrent) -> Mux1/1
  Mux2/1 -> [PhaseCM]
  Mux/1 -> [PhaseAM]
  [PhaseAM] -> PhaseAM/1
  [PhaseBM] -> PhaseBM/1
  [PhaseCM] -> PhaseCM/1
  connections:
  PhaseM1/RConn2 -- N/RConn1 -- Resistor/LConn1 -- PhaseM2/RConn2 -- PhaseM/RConn2
  PhaseM2/RConn1 -- PhaseOutC/RConn1
  PhaseM/RConn1 -- PhaseOutA/RConn1
  PhaseM1/RConn1 -- PhaseOutB/RConn1
  PhaseM/LConn1 -- PhaseInputA/RConn1
  PhaseM2/LConn1 -- PhaseInputC/RConn1
  PhaseM1/LConn1 -- PhaseInputB/RConn1
  Resistor/RConn1 -- GND/RConn1

== system BLAC_MotorCtrl_Math/Hardware_Sim/VbusSample_Sim ==
  Vbus_Sample_Trigger : Inport
  ADCSample_Sim : Subsystem
  ADCSample_Sim1 : Subsystem
  Add1 : Sum
  Add2 : Sum
  Band-Limited White Noise : simulink/Sources/Band-Limited White Noise  Cov=MC_Sim_NoisePower_VACbus  Ts=MC_Sim_BaseStep  seed=[23222]
  Band-Limited White Noise1 : simulink/Sources/Band-Limited White Noise  Cov=MC_Sim_NoisePower_VDCbus  Ts=MC_Sim_BaseStep  seed=[23241]
  Series RLC Branch : spsSeriesRLCBranchLib/Series RLC Branch  LConnTagsString=__new0  RConnTagsString=__new0  BranchType=R  Resistance=1e3  Inductance=1e-3  SetiL0=off  InitialCurrent=0  Capacitance=1e-6  Setx0=off  InitialVoltage=0  Measurements=None
  Series RLC Branch1 : spsSeriesRLCBranchLib/Series RLC Branch  LConnTagsString=__new0  RConnTagsString=__new0  BranchType=R  Resistance=1e3  Inductance=1e-3  SetiL0=off  InitialCurrent=0  Capacitance=1e-6  Setx0=off  InitialVoltage=0  Measurements=None
  Voltage Measurement : spsVoltageMeasurementLib/Voltage Measurement  PhasorSimulation=off  OutputType=Complex  PSBequivalent=0
  Voltage Measurement1 : spsVoltageMeasurementLib/Voltage Measurement  PhasorSimulation=off  OutputType=Complex  PSBequivalent=0
  DCH : PMIOPort  Side=Left
  DCL : PMIOPort  Port=2  Side=Left
  ACH : PMIOPort  Port=3  Side=Left
  ACL : PMIOPort  Port=4  Side=Left
  Vbus_Sample_AC : Outport
  Vbus_Sample_DC : Outport  Port=2
  wires:
  ADCSample_Sim/1(Sample_Out) -> Vbus_Sample_AC/1
  ADCSample_Sim1/1(Sample_Out) -> Vbus_Sample_DC/1
  Vbus_Sample_Trigger/1 -> ADCSample_Sim1/Trigger, ADCSample_Sim/Trigger
  Band-Limited White Noise/1 -> Add1/2
  Add1/1 -> ADCSample_Sim/1(Sample_In)
  Voltage Measurement/1 -> Add1/1
  Band-Limited White Noise1/1 -> Add2/2
  Voltage Measurement1/1 -> Add2/1
  Add2/1 -> ADCSample_Sim1/1(Sample_In)
  connections:
  ACH/RConn1 -- Voltage Measurement/LConn1 -- Series RLC Branch/LConn1
  ACL/RConn1 -- Voltage Measurement/LConn2 -- Series RLC Branch/RConn1
  DCL/RConn1 -- Series RLC Branch1/RConn1 -- Voltage Measurement1/LConn2
  DCH/RConn1 -- Series RLC Branch1/LConn1 -- Voltage Measurement1/LConn1

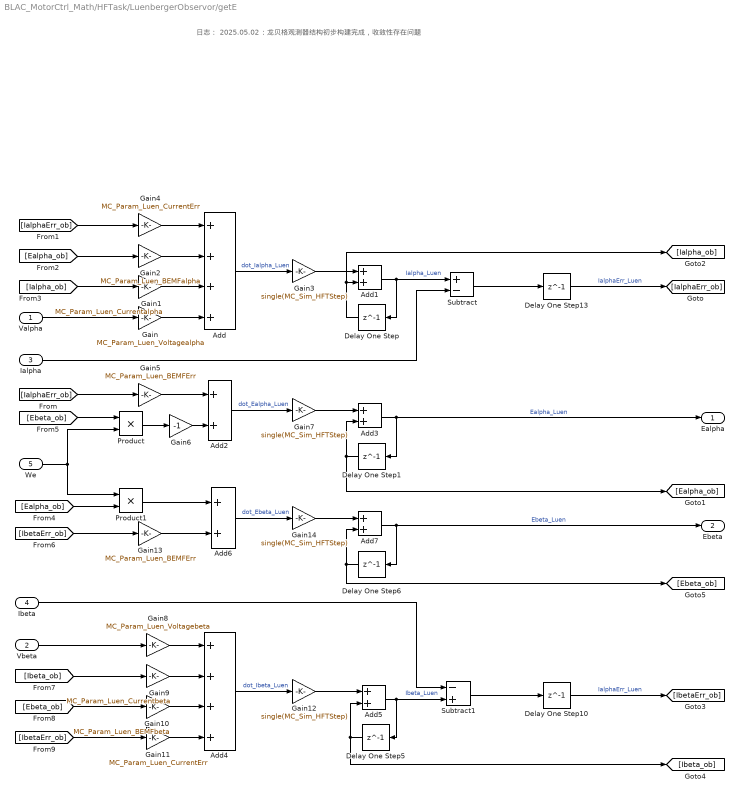
== system BLAC_MotorCtrl_Math/HFTask/LuenbergerObservor/getE ==
  note: 日志：
      | 2025.05.02：龙贝格观测器结构初步构建完成，收敛性存在问题
  Valpha : Inport
  Vbeta : Inport  Port=2
  Ialpha : Inport  Port=3
  Ibeta : Inport  Port=4
  We : Inport  Port=5
  Add : Sum  Inputs=++++
  Add{1..3,5..7} (6 alike) : Sum
  Add4 : Sum  Inputs=++++
  Delay One Step{,1,5..6,10,13} (6 alike) : Delay  DelayLength=1
  Gain : Gain  Gain=MC_Param_Luen_Voltagealpha
  Gain1 : Gain  Gain=MC_Param_Luen_Currentalpha
  Gain10 : Gain  Gain=MC_Param_Luen_BEMFbeta
  Gain11 : Gain  Gain=MC_Param_Luen_CurrentErr
  Gain{3,7,12,14} (4 alike) : Gain  Gain=single(MC_Sim_HFTStep)
  Gain13 : Gain  Gain=MC_Param_Luen_BEMFErr
  Gain2 : Gain  Gain=MC_Param_Luen_BEMFalpha
  Gain4 : Gain  Gain=MC_Param_Luen_CurrentErr
  Gain5 : Gain  Gain=MC_Param_Luen_BEMFErr
  Gain6 : Gain  Gain=-1
  Gain8 : Gain  Gain=MC_Param_Luen_Voltagebeta
  Gain9 : Gain  Gain=MC_Param_Luen_Currentbeta
  Product : Product
  Product1 : Product
  Subtract : Sum  Inputs=+-
  Subtract1 : Sum  Inputs=-+
  Ealpha : Outport
  Ebeta : Outport  Port=2
  wires:
  Valpha/1 -> Gain/1
  Add/1 -> Gain3/1  "dot_Ialpha_Luen"
  Gain2/1 -> Add/2
  Gain1/1 -> Add/3
  Gain/1 -> Add/4
  Gain4/1 -> Add/1
  Gain3/1 -> Add1/1
  Add1/1 -> Subtract/1, Delay One Step/1  "Ialpha_Luen"
  Delay One Step/1 -> [Ialpha_ob], Add1/2
  Ialpha/1 -> Subtract/2
  Subtract/1 -> Delay One Step13/1
  [IalphaErr_ob] -> Gain5/1
  Gain5/1 -> Add2/1
  Gain6/1 -> Add2/2
  Add2/1 -> Gain7/1  "dot_Ealpha_Luen"
  Delay One Step1/1 -> Add3/2, [Ealpha_ob]
  Add3/1 -> Ealpha/1, Delay One Step1/1  "Ealpha_Luen"
  Gain7/1 -> Add3/1
  Product/1 -> Gain6/1
  We/1 -> Product/2, Product1/1
  Vbeta/1 -> Gain8/1
  Gain8/1 -> Add4/1
  Gain9/1 -> Add4/2
  Gain10/1 -> Add4/3
  Gain11/1 -> Add4/4
  [IalphaErr_ob] -> Gain4/1
  [Ealpha_ob] -> Gain2/1
  [Ialpha_ob] -> Gain1/1
  Add4/1 -> Gain12/1  "dot_Ibeta_Luen"
  Delay One Step5/1 -> Add5/2, [Ibeta_ob]
  Add5/1 -> Subtract1/2, Delay One Step5/1  "Ibeta_Luen"
  Gain12/1 -> Add5/1
  Ibeta/1 -> Subtract1/1
  Subtract1/1 -> Delay One Step10/1
  Add6/1 -> Gain14/1  "dot_Ebeta_Luen"
  Gain13/1 -> Add6/2
  Product1/1 -> Add6/1
  Gain14/1 -> Add7/1
  Add7/1 -> Ebeta/1, Delay One Step6/1  "Ebeta_Luen"
  Delay One Step6/1 -> Add7/2, [Ebeta_ob]
  [Ealpha_ob] -> Product1/2
  [Ebeta_ob] -> Product/1
  [IbetaErr_ob] -> Gain13/1
  [Ibeta_ob] -> Gain9/1
  [IbetaErr_ob] -> Gain11/1
  [Ebeta_ob] -> Gain10/1
  Delay One Step13/1 -> [IalphaErr_ob]  "IalphaErr_Luen"
  Delay One Step10/1 -> [IbetaErr_ob]  "IalphaErr_Luen"

== system BLAC_MotorCtrl_Math/HFTask/LuenbergerObservor/getSpeedandTheta ==
  note: 日志：
      | 2025.03.19：反电势正负号识别错误，改正后可以使用
  Ealpha : Inport
  Ebeta : Inport  Port=2
  Add : Sum
  Add1 : Sum
  Add2 : Sum
  Constant : Constant  Value=2*pi  OutDataTypeStr=single
  Delay One Step : Delay  DelayLength=1
  Delay One Step2 : Delay  DelayLength=1
  Gain1 : Gain  Gain=MC_Param_Luen_PLL_Kp
  Gain2 : Gain  Gain=MC_Param_Luen_PLL_Ki
  Gain3 : Gain  Gain=MC_Param_SpeedtoTheta
  Gain5 : Gain  Gain=30/(pi*MC_Motor_Rotor_Pn)  OutDataTypeStr=single  RndMeth=Simplest
  Mod : Math  Operator=mod
  Product : Product
  Product1 : Product
  Sin : Trigonometry  OutputSignalType=real
  Sin1 : Trigonometry  Operator=cos  OutputSignalType=real
  Subtract : Sum  Inputs=+-
  Speed : Outport
  Theta : Outport  Port=2
  We : Outport  Port=3
  wires:
  Gain5/1 -> Speed/1  "SpeedLuen_RPM"
  Product1/1 -> Subtract/2  "LuenCos"
  Product/1 -> Subtract/1  "LuenSin"
  [Theta_Last] -> Sin/1, Sin1/1
  Add1/1 -> We/1, Gain3/1, Gain5/1  "WeLuen"
  Mod/1 -> Delay One Step2/1, Theta/1  "ThetaLuen"
  Delay One Step2/1 -> [Theta_Last], Add2/2
  Constant/1 -> Mod/2
  Add2/1 -> Mod/1
  Gain3/1 -> Add2/1
  Subtract/1 -> Gain1/1, Gain2/1  "LuenErr"
  Gain1/1 -> Add1/1
  Delay One Step/1 -> Add/2
  Add/1 -> Add1/2, Delay One Step/1
  Gain2/1 -> Add/1
  Sin/1 -> Product1/2
  Sin1/1 -> Product/2
  Ealpha/1 -> Product1/1
  Ebeta/1 -> Product/1

== system BLAC_MotorCtrl_Math/HFTask/currentADRC/LESO ==
  Id : Inport
  Ud : Inport  Port=2
  Iq : Inport  Port=3
  Uq : Inport  Port=4
  Add1 : Sum  Inputs=+++  AccumDataTypeStr=single  RndMeth=Simplest
  Add{2,4..6} (4 alike) : Sum
  Add3 : Sum  Inputs=+++  AccumDataTypeStr=single  RndMeth=Simplest
  Delay{,1..3} (4 alike) : Delay  DelayLength=1  InitialCondition=single(0)
  Gain1 : Gain  Gain=2*pi*100*2*pi*100
  Gain2 : Gain  Gain=2*2*pi*100
  Gain4 : Gain  Gain=2*pi*100*2*pi*100
  Gain5 : Gain  Gain=2*2*pi*100
  Gain6 : Gain  Gain=1/single(MC_Motor_Stator_Ld)
  Gain7 : Gain  Gain=1/single(MC_Motor_Stator_Lq)
  Subtract1 : Sum  Inputs=+-
  Subtract2 : Sum  Inputs=+-
  Ts{1..4} (4 alike) : Gain  Gain=single(MC_Sim_HFTStep)  ParamDataTypeStr=single  OutDataTypeStr=single  RndMeth=Simplest
  falFunc : Subsystem  Commented=on
  Id_ESO : Outport
  Iq_ESO : Outport  Port=2
  Id_Dis : Outport  Port=3
  Iq_Dis : Outport  Port=4
  wires:
  [Id_ESO_Delay] -> Subtract1/2
  Id/1 -> Subtract1/1
  Gain2/1 -> Add3/2
  Ud/1 -> Gain6/1
  Add3/1 -> Ts1/1
  Ts1/1 -> Add4/1
  Add4/1 -> Delay/1, Id_ESO/1  "Id_ESO"
  Delay/1 -> Add4/2, [Id_ESO_Delay]
  Subtract1/1 -> Gain1/1, Gain2/1
  Add5/1 -> Id_Dis/1, Delay1/1  "Id_Dis"
  Gain1/1 -> Ts2/1
  Ts2/1 -> Add5/1
  Delay1/1 -> Add3/3, Add5/2
  Delay3/1 -> Add1/3, Add6/2
  Ts4/1 -> Add6/1
  Gain4/1 -> Ts4/1
  Add6/1 -> Iq_Dis/1, Delay3/1  "Iq_Dis"
  Subtract2/1 -> Gain4/1, Gain5/1
  Delay2/1 -> [Iq_ESO_Delay], Add2/2
  Add2/1 -> Iq_ESO/1, Delay2/1  "Iq_ESO"
  Ts3/1 -> Add2/1
  Add1/1 -> Ts3/1
  Uq/1 -> Gain7/1
  Gain5/1 -> Add1/2
  Iq/1 -> Subtract2/1
  [Iq_ESO_Delay] -> Subtract2/2
  Gain6/1 -> Add3/1  "bUd"
  Gain7/1 -> Add1/1  "bUq"

== system BLAC_MotorCtrl_Math/HFTask/currentADRC/NLSEF ==
  Id_Ref : Inport
  Iq_Ref : Inport  Port=2
  Id_ESO : Inport  Port=3
  Iq_ESO : Inport  Port=4
  Id_ESO_Dis : Inport  Port=5
  Iq_ESO_Dis : Inport  Port=6
  Gain1 : Gain  Gain=0.1  OutDataTypeStr=single  RndMeth=Simplest
  Gain2 : Gain  Gain=0.1  OutDataTypeStr=single  RndMeth=Simplest
  Gain3 : Gain  Gain=single(MC_Motor_Stator_Ld)  OutDataTypeStr=single  RndMeth=Simplest
  Gain5 : Gain  Gain=single(MC_Motor_Stator_Lq)  OutDataTypeStr=single  RndMeth=Simplest
  Saturation : Saturate  UpperLimit=MC_Param_CurrentPI_UdMax  LowerLimit=MC_Param_CurrentPI_UdMin
  Saturation1 : Saturate  UpperLimit=MC_Param_CurrentPI_UqMax  LowerLimit=MC_Param_CurrentPI_UqMin
  Subtract : Sum  Inputs=+-
  Subtract1 : Sum  Inputs=+-  OutDataTypeStr=single  AccumDataTypeStr=single  RndMeth=Simplest
  Subtract2 : Sum  Inputs=+-
  Subtract3 : Sum  Inputs=+-
  Ud_ADRC : Outport
  Uq_ADRC : Outport  Port=2
  wires:
  Id_Ref/1 -> Subtract/1
  Id_ESO/1 -> Subtract/2
  Subtract2/1 -> Saturation/1  "Ud_ADRC"
  Saturation/1 -> Ud_ADRC/1
  Saturation1/1 -> Uq_ADRC/1
  Subtract3/1 -> Saturation1/1  "Uq_ADRC"
  Iq_ESO/1 -> Subtract1/2
  Iq_Ref/1 -> Subtract1/1
  Id_ESO_Dis/1 -> Gain3/1
  Gain3/1 -> Subtract2/2
  Iq_ESO_Dis/1 -> Gain5/1
  Gain5/1 -> Subtract3/2
  Gain2/1 -> Subtract3/1
  Subtract/1 -> Gain1/1  "Id_Err"
  Gain1/1 -> Subtract2/1
  Subtract1/1 -> Gain2/1  "Iq_Err"

== system BLAC_MotorCtrl_Math/HFTask/currentPIRControl/currentRController_D ==
  CurrErr : Inport
  Wm : Inport  Port=2
  UReal : Inport  Port=3
  Add : Sum  Inputs=+---
  Delay One Step : Delay  DelayLength=1  InitialCondition=single(0)
  Delay One Step1 : Delay  InitialCondition=single(0)
  Delay One Step2 : Delay  InitialCondition=single(0)
  Gain{,1..3} (4 alike) : Gain
  Saturation : Saturate
  Terminator : Terminator
  Terminator1 : Terminator
  UR_Ref : Outport
  wires:
  Gain/1 -> Add/1
  CurrErr/1 -> Delay One Step2/1, Gain/1
  Delay One Step2/1 -> Gain1/1
  Gain1/1 -> Add/2
  Wm/1 -> Terminator/1
  UReal/1 -> Terminator1/1
  Add/1 -> Saturation/1
  Delay One Step/1 -> Gain2/1
  Delay One Step1/1 -> Gain3/1
  Gain3/1 -> Add/4
  Gain2/1 -> Add/3
  Saturation/1 -> Delay One Step/1, Delay One Step1/1, UR_Ref/1

== system BLAC_MotorCtrl_Math/HFTask/currentPIRControl/currentRController_Q ==
  CurrErr : Inport
  Wm : Inport  Port=2
  UReal : Inport  Port=3
  Add : Sum  Inputs=+---
  Delay One Step : Delay  DelayLength=1  InitialCondition=single(0)
  Delay One Step1 : Delay  InitialCondition=single(0)
  Delay One Step2 : Delay  InitialCondition=single(0)
  Gain{,1..3} (4 alike) : Gain
  Saturation : Saturate
  Terminator : Terminator
  Terminator1 : Terminator
  UR_Ref : Outport
  wires:
  Saturation/1 -> UR_Ref/1, Delay One Step1/1, Delay One Step/1
  Gain2/1 -> Add/3
  Gain3/1 -> Add/4
  Delay One Step1/1 -> Gain3/1
  Delay One Step/1 -> Gain2/1
  Add/1 -> Saturation/1
  UReal/1 -> Terminator1/1
  Wm/1 -> Terminator/1
  Gain1/1 -> Add/2
  Delay One Step2/1 -> Gain1/1
  CurrErr/1 -> Gain/1, Delay One Step2/1
  Gain/1 -> Add/1
